simulink model "ex08_udpreceive"  (R2016a)
settings: Solver=FixedStepAuto  StartTime=0.0  StopTime=30.0  RelTol=1e-3
libraries: embdlinuxlib x2
settings Model: SimulationMode=external  Creator=ohori  LastModifiedBy=ohori
settings SolverCC: PositivePriorityOrder=on
settings OptimizationCC: OptimizeModelRefInitCode=on  LifeSpan=1  MaxStackSize=64
settings HardwareCC: ProdBitPerPointer=32  ProdLargestAtomicInteger=Long  ProdLargestAtomicFloat=Double  ProdWordSize=32  ProdHWDeviceType=ARM Compatible->ARM Cortex  UseEmbeddedCoderFeatures=off  UseSimulinkCoderFeatures=off
settings RTWCC: SystemTargetFile=ert.tlc  HardwareBoard=Raspberry Pi  TemplateMakefile=ert_default_tmf  RTWVerbose=off  Toolchain=GNU GCC Raspberry Pi  IncludeHyperlinkInReport=on
settings CodeAppCC: ForceParamTrailComments=on  OperatorAnnotations=on  SimulinkDataObjDesc=on  SFDataObjDesc=on  MATLABFcnDesc=on  MangleLength=10  InsertBlockDesc=on  MATLABSourceComments=on
settings ERTTargetCC: SupportNonInlinedSFcns=on  SupportVariableSizeSignals=on  ExtMode=on  ExtModeMexArgs='169.254.0.2' 0 17725  ERTSrcFileBannerTemplate=codertarget_code_template.cgt  ERTHdrFileBannerTemplate=codertarget_code_template.cgt  ERTDataSrcFileTemplate=codertarget_code_template.cgt  ERTDataHdrFileTemplate=codertarget_code_template.cgt

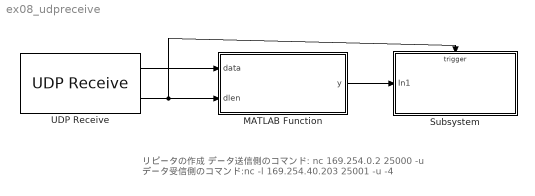
== system ex08_udpreceive ==
  note: リピータの作成
      | データ送信側のコマンド: nc 169.254.0.2 25000 -u
      | データ受信側のコマンド:nc -l 169.254.40.203 25001 -u -4
  MATLAB Function : MATLAB Function  TreatAsAtomicUnit=on
  Subsystem : Subsystem
  UDP Receive : embdlinuxlib/UDP Receive  localURL='0.0.0.0'  localPort=25000  remoteURL='0.0.0.0'  remotePort=-1  recvBufferSize=8192  signalDatatype=uint8  dims=255  isVarSize=off  showBlockingTime=off  blockingTime=0  sampletime=0.01  blockPlatform=Raspberry Pi
  wires:
  UDP Receive/2 -> MATLAB Function/2(dlen), Subsystem/Trigger
  MATLAB Function/1(y) -> Subsystem/1(In1)
  UDP Receive/1 -> MATLAB Function/1(data)

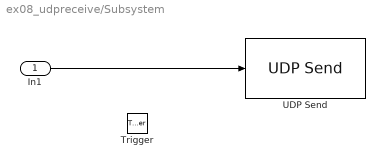
== system ex08_udpreceive/Subsystem ==
  In1 : Inport
  Trigger : TriggerPort  VariantControl=Variant  PortDimensions=1
  UDP Send : embdlinuxlib/UDP Send  remoteURL='169.254.40.203'  remotePort=25001  localURL='255.255.255.255'  localPortSource=Automatically determine  localPort=-1  sampletime=-1  blockPlatform=Raspberry Pi  separateLengthPort=0
  wires:
  In1/1 -> UDP Send/1

== matlab function ex08_udpreceive/MATLAB Function ==
  data: data input; y output; dlen input
function y = fcn(data, dlen)
%#codegen

tmp = char(data)';
out = tmp;

if(dlen>0)
    ds1 = length(tmp) - dlen;
    out = tmp(1,1:dlen);
    out = [out, zeros(1,ds1)];
end

out = int8(out')';

y = out(1:length(data));
